simulink model "PV_MPPT_GRID"  (R2020a)
settings: Solver=FixedStepAuto  StartTime=0.0  StopTime=20  FixedStep=Tss  RelTol=1e-3
values from neighbouring files (symbols this model uses):
  Crc1 = 100e-6    (= 0.0001)    [PV_MPPT_Grid.m]
  f = 50    [PV_MPPT_Grid.m]
  Ki_pid1 = 1    [PV_MPPT_Grid.m]
  Kp_pid1 = .005    (= 0.005)    [PV_MPPT_Grid.m]
  Lf = ((0.1*U^2)/(2*pi*f*Pmin))    (= 0.00612852634199)    [PV_MPPT_Grid.m]
  lower_limit_pid1 = -1.1    [PV_MPPT_Grid.m]
  RLf = Lf*25    (= 0.15321315855)    [PV_MPPT_Grid.m]
  Rrc1 = 1e-3    (= 0.001)    [PV_MPPT_Grid.m]
  Tpid1 = 10*Tss    (= 1e-05)    [PV_MPPT_Grid.m]
  Tss = 10^-6    (= 1e-06)    [PV_MPPT_Grid.m]
  U = 380    [PV_MPPT_Grid.m]
  Upper_limit_pid1 = 1.2    [PV_MPPT_Grid.m]
  Upper_limit_pid2 = 1.1    [PV_MPPT_Grid.m]
undefined symbols (not defined in the file or in its folder): sigbuilder_block
libraries: powerlib x7, powerlib_meascontrol x6, simulink x2, re_lib x1
settings Model: Creator=Junaed  LastModifiedBy=Junaed

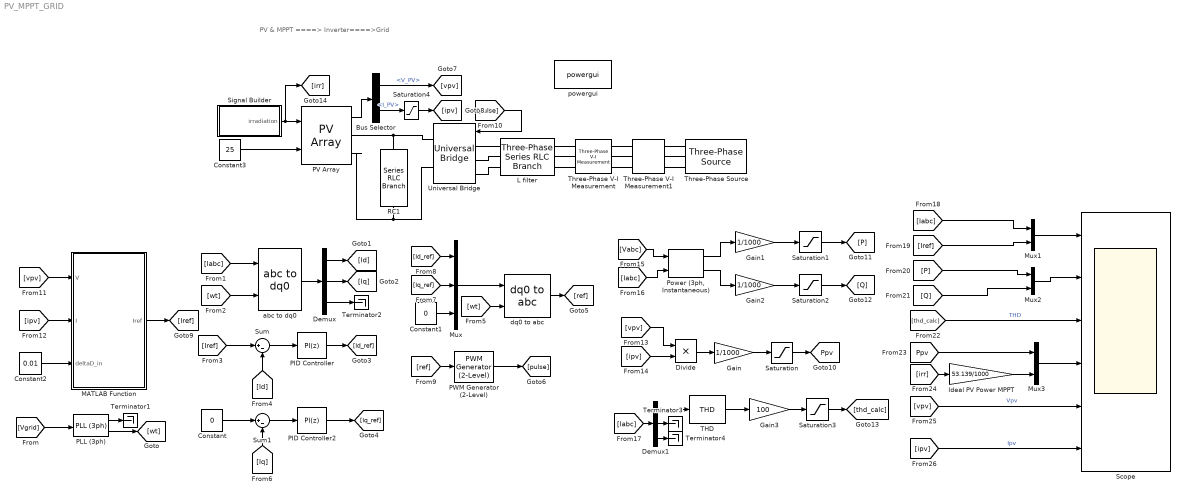
== system PV_MPPT_GRID ==
  note: PV & MPPT ====> Inverter====>Grid
  " RC1" : powerlib/Elements/Series RLC Branch  LConnTagsString=__new0  RConnTagsString=__new0  BranchType=RC  Resistance=Rrc1  Inductance=1e-3  SetiL0=off  InitialCurrent=0  Capacitance=Crc1  Setx0=off  InitialVoltage=0  Measurements=None
  Bus Selector : BusSelector  OutputSignals=V_PV,I_PV
  Constant : Constant  Value=0
  Constant1 : Constant  Value=0
  Constant2 : Constant  Value=0.01
  Constant3 : Constant  Value=25
  Demux : Demux  Outputs=3
  Demux1 : Demux  Outputs=3
  Divide : Product  Inputs=**  RndMeth=Zero  SaturateOnIntegerOverflow=on
  Gain : Gain  Gain=1/1000
  Gain1 : Gain  Gain=1/1000
  Gain2 : Gain  Gain=1/1000
  Gain3 : Gain  Gain=100
  Ideal PV Power MPPT : Gain  Gain=53.139/1000
  L filter : powerlib/Elements/Three-Phase Series RLC Branch  LConnTagsString=A|B|C  RConnTagsString=A|B|C  BranchType=RL  Resistance=RLf  Inductance=Lf  Capacitance=1e-6  Measurements=None
  MATLAB Function : MATLAB Function  TreatAsAtomicUnit=on
  Mux : Mux  Inputs=3
  Mux1 : Mux  Inputs=2
  Mux2 : Mux  Inputs=2
  Mux3 : Mux  Inputs=2
  PID Controller : simulink/Continuous/PID Controller  Controller=PI  Form=Parallel  TimeDomain=Discrete-time  UseExternalTs=off  SampleTime=Tpid1  IntegratorMethod=Forward Euler  FilterMethod=Forward Euler  ControllerParametersSource=internal  P=Kp_pid1  I=Ki_pid1  D=0  UseFilter=on  N=100  TunerSelectOption=Transfer Function Based (PID Tuner App)  InitialConditionSource=internal  InitialConditionForIntegrator=0  InitialConditionForFilter=0  DifferentiatorICPrevScaledInput=0  ExternalReset=none  TrackingMode=off  Kt=1  LimitOutput=on  UpperSaturationLimit=Upper_limit_pid1  LowerSaturationLimit=lower_limit_pid1  LinearizeAsGain=on  AntiWindupMode=none  Kb=1  POutMin=[]  POutMax=[]  IOutMin=[]  IOutMax=[]  DOutMin=[]  DOutMax=[]  NOutMin=[]  NOutMax=[]  SumOutMin=[]  SumOutMax=[]  SaturationOutMin=[]  SaturationOutMax=[]  PParamMin=[]  PParamMax=[]  IParamMin=[]  IParamMax=[]  DParamMin=[]  DParamMax=[]  NParamMin=[]  NParamMax=[]  KbParamMin=[]  KbParamMax=[]  KtParamMin=[]  KtParamMax=[]  KbOutMin=[]  KbOutMax=[]  KtOutMin=[]  KtOutMax=[]  IntegratorOutMin=[]  IntegratorOutMax=[]  FilterOutMin=[]  FilterOutMax=[]  SumI1OutMin=[]  SumI1OutMax=[]  SumI2OutMin=[]  SumI2OutMax=[]  SumI3OutMin=[]  SumI3OutMax=[]  SumI4OutMin=[]  SumI4OutMax=[]  SumDOutMin=[]  SumDOutMax=[]  DifferentiatorOutMin=[]  DifferentiatorOutMax=[]  FilterDiffOutCoefMin=[]  FilterDiffOutCoefMax=[]  ReciprocalOutMin=[]  ReciprocalOutMax=[]  SumDenOutMin=[]  SumDenOutMax=[]  SumNumOutMin=[]  SumNumOutMax=[]  DivideOutMin=[]  DivideOutMax=[]  UdiffTsProdOutMin=[]  UdiffTsProdOutMax=[]  NTsProdOutMin=[]  NTsProdOutMax=[]  UintegralTsProdOutMin=[]  UintegralTsProdOutMax=[]  UngainTsProdOutMin=[]  UngainTsProdOutMax=[]  IntegratorContinuousStateAttributes=''  IntegratorStateMustResolveToSignalObject=off  IntegratorRTWStateStorageClass=Auto  FilterContinuousStateAttributes=''  FilterStateMustResolveToSignalObject=off  FilterRTWStateStorageClass=Auto  ParallelPVariant=InternalParameters  IdealPVariant=Disabled  IVariant=InternalParameters  DVariant=Disabled  IntegratorVariant=Discrete  SatVariant=Enabled  AWVariant=Passthrough  PCopyVariant=Disabled  TRVariant=Disabled  FdbkBlocksVariant=Forward  IdealPFdbkVariant=Disabled  SatFdbkVariant=Disabled  DerivativeFilterVariant=Disabled  NVariant=Disabled  NCopyVariant=Disabled_SignalSpec  FilterICVariant=Disabled  IntegratorICVariant=InternalICs  ExternalResetVariant=Disabled  TRSumVariant=Passthrough  SumFdbkVariant=Disabled  SumVariant=Sum_PI  TsampFilterVariant=InternalTs  TsampNgainVariant=Passthrough  TsampIntegralVariant=Passthrough
  PID Controller2 : simulink/Continuous/PID Controller  Controller=PI  Form=Parallel  TimeDomain=Discrete-time  UseExternalTs=off  SampleTime=Tpid1  IntegratorMethod=Forward Euler  FilterMethod=Forward Euler  ControllerParametersSource=internal  P=Kp_pid1  I=Ki_pid1  D=0  UseFilter=on  N=100  TunerSelectOption=Transfer Function Based (PID Tuner App)  InitialConditionSource=internal  InitialConditionForIntegrator=0  InitialConditionForFilter=0  DifferentiatorICPrevScaledInput=0  ExternalReset=none  TrackingMode=off  Kt=1  LimitOutput=on  UpperSaturationLimit=Upper_limit_pid2  LowerSaturationLimit=0  LinearizeAsGain=on  AntiWindupMode=none  Kb=1  POutMin=[]  POutMax=[]  IOutMin=[]  IOutMax=[]  DOutMin=[]  DOutMax=[]  NOutMin=[]  NOutMax=[]  SumOutMin=[]  SumOutMax=[]  SaturationOutMin=[]  SaturationOutMax=[]  PParamMin=[]  PParamMax=[]  IParamMin=[]  IParamMax=[]  DParamMin=[]  DParamMax=[]  NParamMin=[]  NParamMax=[]  KbParamMin=[]  KbParamMax=[]  KtParamMin=[]  KtParamMax=[]  KbOutMin=[]  KbOutMax=[]  KtOutMin=[]  KtOutMax=[]  IntegratorOutMin=[]  IntegratorOutMax=[]  FilterOutMin=[]  FilterOutMax=[]  SumI1OutMin=[]  SumI1OutMax=[]  SumI2OutMin=[]  SumI2OutMax=[]  SumI3OutMin=[]  SumI3OutMax=[]  SumI4OutMin=[]  SumI4OutMax=[]  SumDOutMin=[]  SumDOutMax=[]  DifferentiatorOutMin=[]  DifferentiatorOutMax=[]  FilterDiffOutCoefMin=[]  FilterDiffOutCoefMax=[]  ReciprocalOutMin=[]  ReciprocalOutMax=[]  SumDenOutMin=[]  SumDenOutMax=[]  SumNumOutMin=[]  SumNumOutMax=[]  DivideOutMin=[]  DivideOutMax=[]  UdiffTsProdOutMin=[]  UdiffTsProdOutMax=[]  NTsProdOutMin=[]  NTsProdOutMax=[]  UintegralTsProdOutMin=[]  UintegralTsProdOutMax=[]  UngainTsProdOutMin=[]  UngainTsProdOutMax=[]  IntegratorContinuousStateAttributes=''  IntegratorStateMustResolveToSignalObject=off  IntegratorRTWStateStorageClass=Auto  FilterContinuousStateAttributes=''  FilterStateMustResolveToSignalObject=off  FilterRTWStateStorageClass=Auto  ParallelPVariant=InternalParameters  IdealPVariant=Disabled  IVariant=InternalParameters  DVariant=Disabled  IntegratorVariant=Discrete  SatVariant=Enabled  AWVariant=Passthrough  PCopyVariant=Disabled  TRVariant=Disabled  FdbkBlocksVariant=Forward  IdealPFdbkVariant=Disabled  SatFdbkVariant=Disabled  DerivativeFilterVariant=Disabled  NVariant=Disabled  NCopyVariant=Disabled_SignalSpec  FilterICVariant=Disabled  IntegratorICVariant=InternalICs  ExternalResetVariant=Disabled  TRSumVariant=Passthrough  SumFdbkVariant=Disabled  SumVariant=Sum_PI  TsampFilterVariant=InternalTs  TsampNgainVariant=Passthrough  TsampIntegralVariant=Passthrough
  PLL (3ph) : powerlib_meascontrol/PLL/PLL (3ph)  Fmin=45  Par_Init=[0, 50]  ParK=[180, 3200, 1]  TcD=1e-4  MaxRateChangeFreq=12  FilterCutOffFreq=25  Ts=Tss  AGC=on
  PV Array : re_lib/Solar/PV Array  Npar=Parallel_strings  Nser=Series_connected_modules_per_string  PlotType=array @ 1000 W/m2 & specified temperatures  S_vec="[ 1000  500  100 ]"  Temp_C_vec="[ 45 25  ]"  ModuleName=SunPower SPR-230-WHT-U  PlotWhenSelected=off  Pm=230.01  Ncell=72  Voc=48.7  Isc=5.99  Vm=41  Im=5.61  beta_Voc_pc=-0.28209  alpha_Isc_pc=0.035593  beta_Voc=-0.13738  alpha_Isc=0.002132  IL=5.997  I0=9.233e-12  nI=0.96882  Rsh=320.7087  Rs=0.36905  RobustModel=off  RobustCellTemperature=25  BAL=on  Tc=1e-6  Tfilter=5e-5
  PWM Generator (2-Level) : powerlib_meascontrol/Pulse & Signal Generators/PWM Generator (2-Level)  ModulatorType=Three-phase bridge (6 pulses)  ModulatorMode=Unsynchronized  Fc=fsw  Pc=90  nF=27  MinMax="[ -1  1 ]"  SamplingTechnique=Natural  ModulatingSignals=off  m=0.8  Freq=60  Phase=0  Ts=Tss  ShowCarrierOutport=off
  "Power (3ph, Instantaneous)" : powerlib_meascontrol/Measurements/Power (3ph, Instantaneous)
  Saturation{,1..3} (4 alike) : Saturate  UpperLimit=60  LowerLimit=0
  Saturation4 : Saturate  UpperLimit=200  LowerLimit=0
  Scope : Scope  NumInputPorts=6
  Signal Builder : Subsystem  Tag=STV Subsys  LoadFcn=sigbuilder_block('load',[0 30 1024.5 488.25 ]);  StartFcn=sigbuilder_block('start');  StopFcn=sigbuilder_block('stop');  ClipboardFcn=sigbuilder_block('clipboard');  mask(Sigbuilder block){tuvar=[0:10]}
      mask help: Simulink:masks:SigbuilderBlock_MD
      mask init:
      | if ~strcmp(get_param(bdroot(gcbh),'SimulationStatus'),'stopped') tuvar = sigbuilder_block('maskInit'); end
      settings: CopyFcn=sigbuilder_block('copy');  DeleteFcn=sigbuilder_block('delete');  ModelCloseFcn=sigbuilder_block('modelClose');  PreSaveFcn=sigbuilder_block('preSave');  PauseFcn=sigbuilder_block('pause');  ContinueFcn=sigbuilder_block('continue');  NameChangeFcn=sigbuilder_block('namechange');  OpenFcn=sigbuilder_block('open',[437.6 153 550.4 359.25 ]);  CloseFcn=sigbuilder_block('close');
      mask Display: plot(0, 0, 100, 100,[2, 2, 32, 32, 2], [68, 8, 8, 68, 68],[32, 2], [38, 38], [32, 19, 2],[53, 60, 44], [32, 17, 17, 2],[16, 16, 31, 31]);txt = getActiveGroup(gcbh);text(2, 100, txt,'verticalAlignment', 'top');
  Sum : Sum  Inputs=|+-
  Sum1 : Sum  Inputs=|+-
  THD : powerlib_meascontrol/Measurements/THD  Freq=f  Ts=Tss
  Terminator{1..4} (4 alike) : Terminator
  Three-Phase V-I Measurement : powerlib/Measurements/Three-Phase V-I Measurement  VoltageMeasurement=phase-to-ground  SetLabelV=on  LabelV=Vabc  Vpu=off  VpuLL=off  CurrentMeasurement=yes  SetLabelI=on  LabelI=Iabc  Ipu=off  Pbase=100e6  Vbase=500e3  OutputType=Complex  PhasorSimulation=off  PSBequivalent=0
  Three-Phase V-I Measurement1 : powerlib/Measurements/Three-Phase V-I Measurement  VoltageMeasurement=phase-to-ground  SetLabelV=on  LabelV=Vgrid  Vpu=off  VpuLL=off  CurrentMeasurement=yes  SetLabelI=on  LabelI=Igrid  Ipu=off  Pbase=100e6  Vbase=500e3  OutputType=Complex  PhasorSimulation=off  PSBequivalent=0
  Three-Phase Source : powerlib/Electrical Sources/Three-Phase Source  InternalConnection=Yg  VoltagePhases=off  Voltage=U  PhaseAngle=0  Voltage_phases=[25e3 25e3 25e3]/sqrt(3)  PhaseAngles_phases=[0 -120 +120]  Frequency=f  NonIdealSource=on  SpecifyImpedance=on  Resistance=0.8929  Inductance=16.58e-3  ShortCircuitLevel=100e6  BaseVoltage=U  XRratio=7  BusType=swing  Pref=10e3  Qref=0  Prefabc=[10e3, 10e3, 10e3]  Qrefabc=[0, 0, 0]  Qmin=-inf  Qmax=inf
  Universal Bridge : powerlib/Power Electronics/Universal Bridge  Arms=3  SnubberResistance=1e5  SnubberCapacitance=inf  Device=IGBT / Diodes  Ron=1e-3  Lon=0  ForwardVoltages="[  0  0  ]"  ForwardVoltage=0  GTOparameters=[ 10e-6 , 20e-6 ]  IGBTparameters=[ 1e-6 , 2e-6 ]  Measurements=None  Measurements_2=None  converterType=Rectifier
  abc to dq0 : powerlib_meascontrol/Transformations/abc to dq0  Alignment=90 degrees behind phase A axis
  dq0 to abc : powerlib_meascontrol/Transformations/dq0 to abc  Alignment=90 degrees behind phase A axis
  powergui : powerlib/powergui  Priority=1  SimulationMode=Discrete  SampleTime=Tss  frequency=60  Iterations=50  frequencyindice=50  Pbase=100e6  ErrMax=1e-4  UnitsV=kV  UnitsW=MW  buscounter=0  FunctionMessages=off  echomessages=off  EnableUseOfTLC=off  CurrentSourceSwitches=off  DisableSnubberDevices=off  DisableRonSwitches=off  DisableVfSwitches=off  DisplayEquations=off  AutomaticDiscreteSolvers=off  SolverType=Tustin/Backward Euler (TBE)  Interpol=off  ExternalGateDelay=off  methode=off  Ts=100  x0status=blocks  SPID=on  SwTol=0  HookPort=off  NonlinearTolerance=1e-4  nMaxIteration=100  ContinueOnMaxIteration=off  RestoreLinks=warning  ResistiveCurrentMeasurement=off  Frange=[0:2:500]  Ylog=off  Xlog=on  ShowGrid=off  save=off  variable=ZData  structure=0  ZoomFFT=off  StartTime=0.0  cycles=1  DisplayStyle=1  fundamental=60  FreqAxis=off  MaxFrequency=1000  frequencyindicesteady=1  RmsSteady=1  display=off
  tag scope: Ppv=global
  wires:
  [Vgrid] -> PLL (3ph)/1
  PLL (3ph)/2 -> [wt]
  [Iabc] -> abc to dq0/1
  [wt] -> abc to dq0/2
  abc to dq0/1 -> Demux/1
  Demux/1 -> [Id]
  Demux/2 -> [Iq]
  [Iref] -> Sum/1
  [Id] -> Sum/2
  Sum/1 -> PID Controller/1
  PID Controller/1 -> [Id_ref]
  PID Controller2/1 -> [Iq_ref]
  Sum1/1 -> PID Controller2/1
  [Iq] -> Sum1/2
  Constant/1 -> Sum1/1
  Mux/1 -> dq0 to abc/1
  [wt] -> dq0 to abc/2
  [Iq_ref] -> Mux/2
  [Id_ref] -> Mux/1
  Constant1/1 -> Mux/3
  dq0 to abc/1 -> [ref]
  [ref] -> PWM Generator (2-Level)/1
  PWM Generator (2-Level)/1 -> [pulse]
  [pulse] -> Universal Bridge/1
  PV Array/1 -> Bus Selector/1
  Bus Selector/1 -> [vpv]  "<V_PV>"
  Bus Selector/2 -> Saturation4/1  "<I_PV>"
  [vpv] -> MATLAB Function/1(V)
  [ipv] -> MATLAB Function/2(I)
  Constant2/1 -> MATLAB Function/3(deltaD_in)
  MATLAB Function/1(Iref) -> [Iref]
  Signal Builder/1(irradiation) -> [irr], PV Array/1
  Constant3/1 -> PV Array/2
  [vpv] -> Divide/1
  [ipv] -> Divide/2
  Divide/1 -> Gain/1
  Gain/1 -> Saturation/1
  Saturation/1 -> [Ppv]
  [Vabc] -> "Power (3ph, Instantaneous)"/1
  [Iabc] -> "Power (3ph, Instantaneous)"/2
  "Power (3ph, Instantaneous)"/1 -> Gain1/1
  "Power (3ph, Instantaneous)"/2 -> Gain2/1
  Gain1/1 -> Saturation1/1
  Gain2/1 -> Saturation2/1
  Saturation1/1 -> [P]
  Saturation2/1 -> [Q]
  [Iabc] -> Demux1/1
  Demux1/1 -> THD/1
  THD/1 -> Gain3/1
  Gain3/1 -> Saturation3/1
  Saturation3/1 -> [thd_calc]
  Mux1/1 -> Scope/1
  Mux2/1 -> Scope/2
  [Iabc] -> Mux1/1
  [Iref] -> Mux1/2
  [P] -> Mux2/1
  [Q] -> Mux2/2
  [thd_calc] -> Scope/3  "THD"
  [irr] -> Ideal PV Power MPPT/1
  [Ppv] -> Mux3/1
  Mux3/1 -> Scope/4
  Ideal PV Power MPPT/1 -> Mux3/2
  Saturation4/1 -> [ipv]
  [vpv] -> Scope/5  "Vpv"
  [ipv] -> Scope/6  "Ipv"
  PLL (3ph)/1 -> Terminator1/1
  Demux/3 -> Terminator2/1
  Demux1/2 -> Terminator3/1
  Demux1/3 -> Terminator4/1
  connections:
  PV Array/RConn1 -- " RC1"/LConn1 -- Universal Bridge/RConn1
  PV Array/RConn2 -- " RC1"/RConn1 -- Universal Bridge/RConn2
  L filter/LConn1 -- Universal Bridge/LConn1
  Universal Bridge/LConn2 -- L filter/LConn2
  Universal Bridge/LConn3 -- L filter/LConn3
  L filter/RConn1 -- Three-Phase V-I Measurement/LConn1
  L filter/RConn2 -- Three-Phase V-I Measurement/LConn2
  L filter/RConn3 -- Three-Phase V-I Measurement/LConn3
  Three-Phase V-I Measurement1/LConn1 -- Three-Phase Source/RConn1
  Three-Phase V-I Measurement1/LConn2 -- Three-Phase Source/RConn2
  Three-Phase V-I Measurement1/LConn3 -- Three-Phase Source/RConn3
  Three-Phase V-I Measurement/RConn1 -- Three-Phase V-I Measurement1/RConn1
  Three-Phase V-I Measurement/RConn2 -- Three-Phase V-I Measurement1/RConn2
  Three-Phase V-I Measurement/RConn3 -- Three-Phase V-I Measurement1/RConn3

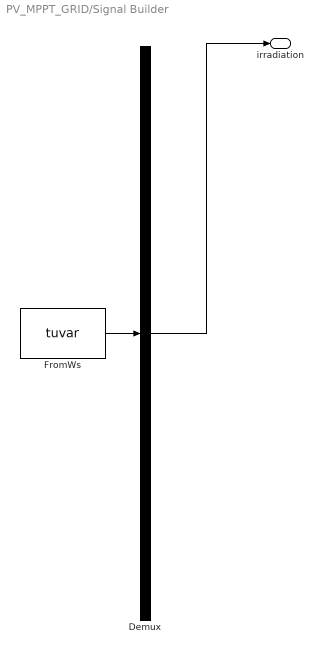
== system PV_MPPT_GRID/Signal Builder ==
  Demux : Demux  Tag=STV Demux  Outputs=1
      settings: DisplayOption=none
  FromWs : FromWorkspace  Tag=STV FromWs  VariableName=tuvar
      SigBuilderData=|
      | common.afterFinalStr = 'Extrapolate'
      | common.sampleTime = 0
      | dataSet.timeRange = [0 20]
      | dataSet.name = 'Mean Irradiation'
      | sbobj.Groups.Name = 'Mean Irradiation'
      | sbobj.Groups.Signals.Name = 'irradiation'
      | sbobj.Groups.Signals.XData = [0 1 2 3 4 5 6 7 8 9 10 11 12 13 14 15 16 17 18 19 20]
      | sbobj.Groups.Signals.YData = [0 0 200 300 400 500 600 700 800 1000 1000 1000 800 700 600 500 400 300 200 0 0]
      | sbobj.Groups.TimeRange = [0 20]
  irradiation : Outport  Tag=STV Outport
  wires:
  FromWs/1 -> Demux/1
  Demux/1 -> irradiation/1

== matlab function PV_MPPT_GRID/MATLAB Function ==
  data: V input; Iref output; I input; deltaD_in input
function Iref = MPPT_Control(V,I,deltaD_in)

Iref_init = 0.1;
I_min = 0;
I_max=150;

persistent Vold Pold Iref_old ;

if isempty(Vold)
    Vold = 0;
    Pold = 0;
    Iref_old = Iref_init;
end
P=V*I;
dV=V-Vold;
dP=P-Pold;
Iref=Iref_old;
deltaD=deltaD_in;

if dP~=0  &&  V>400
    if dP<0
        if dV<0
            Iref = Iref_old-deltaD;
        else
            Iref = Iref_old+deltaD;
        end
    else
        if dV<0
            Iref = Iref_old+deltaD;
        else
            Iref = Iref_old-deltaD;
        end
    end
end
% these are limit the current between minimum and maximum
if Iref >=I_max
    Iref=I_max;
elseif Iref< I_min
    Iref=I_min;
end
Iref_old = Iref;
Vold=V;
Pold=P;
end
